simulink model "RW_MDL"  (R2025b)
settings: Solver=VariableStepAuto  StartTime=0.0  StopTime=24*3600  RelTol=1e-3
values from neighbouring files (symbols this model uses):
  initSatPhiRef = initSatPhiRef * (pi / 180)    (= 0.785398163397)    [input_script.m]
  satPhiRefAngVel = satPhiRefAngVel * (pi / 180)    (= 7.27220521664e-05)    [input_script.m]
  x0 = [initSatPhi; initSatAngVel; initWheelAngVel] .* (pi / 180)    [input_script.m]
libraries: slpidlib x1, simulink x1
settings Model: Creator=antoniohernandez-rodiciomateos  LastModifiedBy=antoniohernandez-rodiciomateos

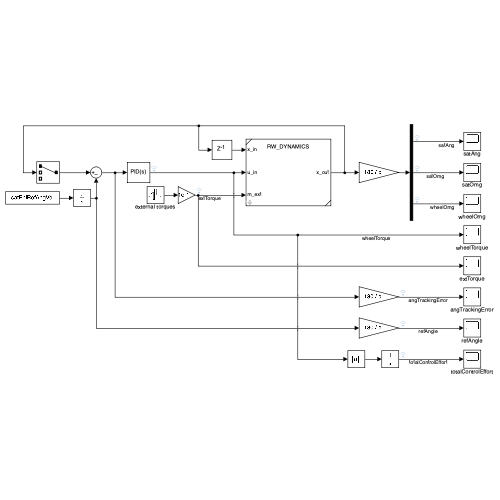
[thumbnail: Simulink's stored preview of the top-level diagram]
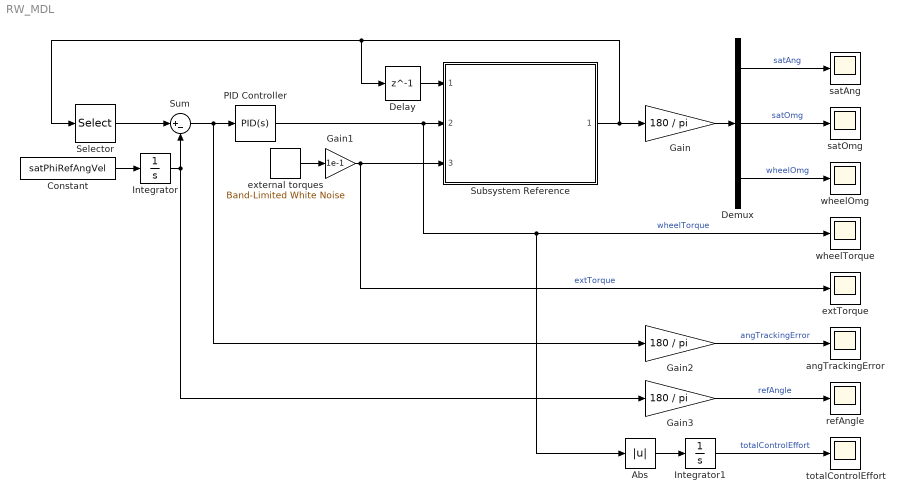
== system RW_MDL ==
  Abs : Abs  SaturateOnIntegerOverflow=off
  Constant : Constant  Value=satPhiRefAngVel
  Delay : Delay  DelayLength=1  InitialCondition=x0
  Demux : Demux  Outputs=3
  Gain : Gain  Gain=180 / pi
  Gain1 : Gain  Gain=1e-1
  Gain2 : Gain  Gain=180 / pi
  Gain3 : Gain  Gain=180 / pi
  Integrator : Integrator  InitialCondition=initSatPhiRef
  Integrator1 : Integrator
  PID Controller : slpidlib/PID Controller  Controller=PID  Form=Parallel  TimeDomain=Continuous-time  UseExternalTs=off  SampleTime=-1  IntegratorMethod=Forward Euler  FilterMethod=Forward Euler  ControllerParametersSource=internal  P=2.84655991347559  I=0.121445412862792  UseKiTs=off  D=16.3465418426238  UseExternalDerivativeSource=off  N=10.4897155810233  UseFilter=on  TunerSelectOption=Transfer Function Based (PID Tuner App)  InitialConditionSource=internal  InitialConditionForIntegrator=0  InitialConditionForFilter=0  DifferentiatorICPrevScaledInput=0  ExternalReset=none  TrackingMode=off  Kt=1  LimitOutput=off  SatLimitsSource=internal  UpperSaturationLimit=inf  LowerSaturationLimit=-inf  LinearizeAsGain=on  AntiWindupMode=none  Kb=1  LimitIntegrator=off  UpperIntegratorSaturationLimit=inf  LowerIntegratorSaturationLimit=-inf  POutMin=[]  POutMax=[]  IOutMin=[]  IOutMax=[]  DOutMin=[]  DOutMax=[]  NOutMin=[]  NOutMax=[]  SumOutMin=[]  SumOutMax=[]  SaturationOutMin=[]  SaturationOutMax=[]  PParamMin=[]  PParamMax=[]  IParamMin=[]  IParamMax=[]  DParamMin=[]  DParamMax=[]  NParamMin=[]  NParamMax=[]  KbParamMin=[]  KbParamMax=[]  KtParamMin=[]  KtParamMax=[]  KbOutMin=[]  KbOutMax=[]  KtOutMin=[]  KtOutMax=[]  IntegratorOutMin=[]  IntegratorOutMax=[]  FilterOutMin=[]  FilterOutMax=[]  SumI1OutMin=[]  SumI1OutMax=[]  SumI2OutMin=[]  SumI2OutMax=[]  SumI3OutMin=[]  SumI3OutMax=[]  SumI4OutMin=[]  SumI4OutMax=[]  SumDOutMin=[]  SumDOutMax=[]  DifferentiatorOutMin=[]  DifferentiatorOutMax=[]  FilterDiffOutCoefMin=[]  FilterDiffOutCoefMax=[]  ReciprocalOutMin=[]  ReciprocalOutMax=[]  SumDenOutMin=[]  SumDenOutMax=[]  SumNumOutMin=[]  SumNumOutMax=[]  DivideOutMin=[]  DivideOutMax=[]  UdiffTsProdOutMin=[]  UdiffTsProdOutMax=[]  NTsProdOutMin=[]  NTsProdOutMax=[]  UintegralTsProdOutMin=[]  UintegralTsProdOutMax=[]  UngainTsProdOutMin=[]  UngainTsProdOutMax=[]  ClampingZeroOutDataTypeStr=Inherit: Inherit via back propagation  ClampingZeroOutMin=[]  ClampingZeroOutMax=[]  FilterDenConstantOutDataTypeStr=Inherit: Inherit via back propagation  FilterDenConstantOutMin=[]  FilterDenConstantOutMax=[]  PCopyOutDataTypeStr=Inherit: Inherit via back propagation  PCopyOutMin=[]  PCopyOutMax=[]  NCopyOutDataTypeStr=Inherit: Inherit via back propagation  NCopyOutMin=[]  NCopyOutMax=[]  IntegratorContinuousStateAttributes=''  IntegratorStateMustResolveToSignalObject=off  IntegratorRTWStateStorageClass=Auto  FilterContinuousStateAttributes=''  FilterStateMustResolveToSignalObject=off  FilterRTWStateStorageClass=Auto  ParallelPVariant=InternalParameters  IdealPVariant=Disabled  IVariant=InternalParameters  DVariant=InternalParameters  IntegratorVariant=Continuous  SatVariant=Disabled  AWVariant=Passthrough  PCopyVariant=Disabled  TRVariant=Disabled  FdbkBlocksVariant=Forward  IdealPFdbkVariant=Disabled  SatFdbkVariant=Disabled  DerivativeFilterVariant=ContFilter  NVariant=InternalParameters  NCopyVariant=Disabled  FilterICVariant=InternalICsFilter  IntegratorICVariant=InternalICs  ExternalResetVariant=Disabled  TRSumVariant=Passthrough  SumFdbkVariant=Disabled  SumVariant=Sum_PID  TsampFilterVariant=InternalTs  TsampNgainVariant=Passthrough  TsampIntegralVariant=Disabled_SignalSpec  ExternalSaturationOutDataTypeStr=Inherit: Same as second input  DerivativeSourceVariant=ErrorSignal  PreIntVariant=InternalPreInt
  Selector : Selector  InputPortWidth=3  IndexOptions=Index vector (dialog)  Indices=[1]  OutputSizes=1
  Subsystem Reference : Subsystem  ReferencedSubsystem=RW_DYNAMICS  Js=satI  Jw=wheelI  x0=x0
  Sum : Sum  Inputs=|+-
  angTrackingError : Scope
      settings: DataLoggingVariableName=ScopeData5
  extTorque : Scope
      settings: DataLoggingVariableName=ScopeData4
  external torques : simulink/Sources/Band-Limited White Noise  Cov=[0.1]  Ts=0.1  seed=[23341]
  refAngle : Scope
      settings: DataLoggingVariableName=ScopeData6
  satAng : Scope
  satOmg : Scope
  totalControlEffort : Scope
      settings: DataLoggingVariableName=ScopeData7
  wheelOmg : Scope
      settings: DataLoggingVariableName=ScopeData2
  wheelTorque : Scope
      settings: DataLoggingVariableName=ScopeData3
  wires:
  Delay/1 -> Subsystem Reference/1
  Subsystem Reference/1 -> Delay/1, Selector/1, Gain/1
  PID Controller/1 -> Subsystem Reference/2, Abs/1, wheelTorque/1  "wheelTorque"
  Gain/1 -> Demux/1
  Demux/1 -> satAng/1  "satAng"
  Demux/2 -> satOmg/1  "satOmg"
  Demux/3 -> wheelOmg/1  "wheelOmg"
  Selector/1 -> Sum/1
  Constant/1 -> Integrator/1
  Sum/1 -> Gain2/1, PID Controller/1
  external torques/1 -> Gain1/1
  Gain1/1 -> Subsystem Reference/3, extTorque/1  "extTorque"
  Integrator/1 -> Gain3/1, Sum/2
  Gain3/1 -> refAngle/1  "refAngle"
  Gain2/1 -> angTrackingError/1  "angTrackingError"
  Integrator1/1 -> totalControlEffort/1  "totalControlEffort"
  Abs/1 -> Integrator1/1
